simulink model "generalizedBiadForcesTest"  (Simulink 7.9)
settings: Solver=FixedStepDiscrete  StartTime=0.0  StopTime=3  FixedStep=1  RelTol=1e-3
settings Model: Creator=jorhabib  LastModifiedBy=jorhabib

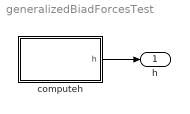
== system generalizedBiadForcesTest ==
  computeh : Subsystem  mask{val=7, robotname='icubSim', localname='simulink'}
      mask prompts: val "Block type"; robotname "Robot name"; localname "Module name"
  h : Outport
  wires:
  computeh/1(h) -> h/1

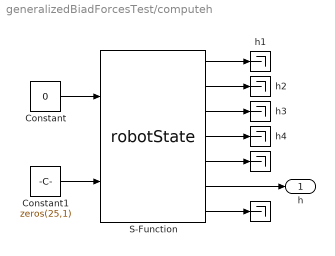
== system generalizedBiadForcesTest/computeh ==
  " " : Terminator
  "  " : Terminator
  Constant : Constant  Value=0  OutDataTypeStr=int8  SampleTime=-1
  Constant1 : Constant  Value=zeros(25,1)  OutDataTypeStr=double  SampleTime=-1
  S-Function : S-Function  FunctionName=robotState  Parameters=7,'icubSim','simulink'  EnableBusSupport=off
  h{1..4} (4 alike) : Terminator
  h : Outport
  wires:
  S-Function/6 -> h/1
  S-Function/7 -> " "/1
  S-Function/5 -> "  "/1
  S-Function/4 -> h4/1
  S-Function/3 -> h3/1
  S-Function/2 -> h2/1
  S-Function/1 -> h1/1
  Constant1/1 -> S-Function/2
  Constant/1 -> S-Function/1
